simulink model "notlin2"  (Simulink 6.2)
settings: Solver=ode45  StartTime=0  StopTime=0.2
libraries: simulink x6
settings Model: Creator=Admin  LastModifiedBy=wahwat
settings OptimizationCC: BooleanDataType=off
settings HardwareCC: TargetUnknown=on

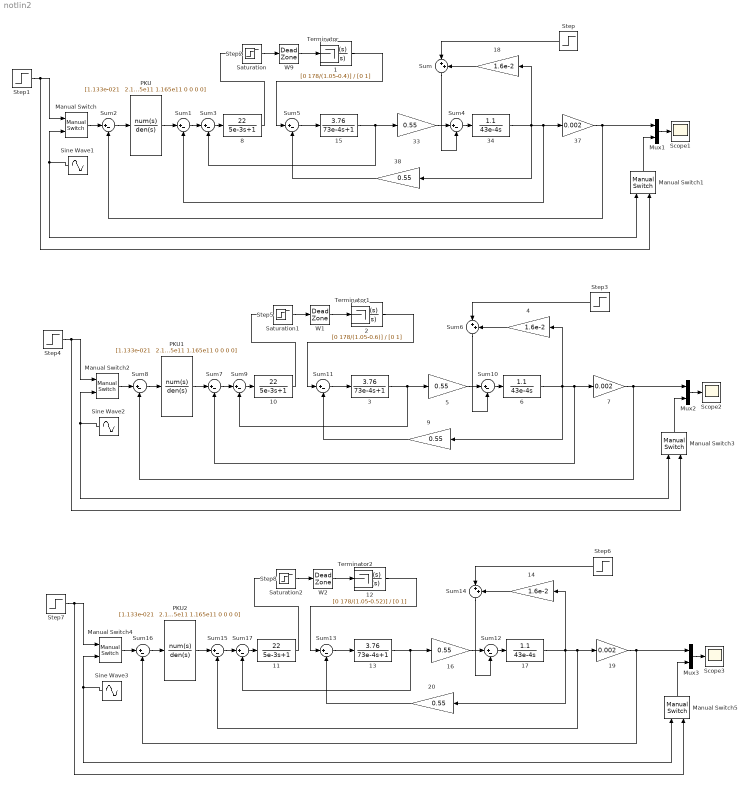
== system notlin2 ==
  1 : TransferFcn  Numerator=[0 178/(1.05-0.4)]  Denominator=[0 1]
  10 : TransferFcn  Numerator=[22]  Denominator=[5e-3 1]
  11 : TransferFcn  Numerator=[22]  Denominator=[5e-3 1]
  12 : TransferFcn  Numerator=[0 178/(1.05-0.52)]  Denominator=[0 1]
  13 : TransferFcn  Numerator=[3.76]  Denominator=[73e-4 1]
  14 : Gain  Orientation=left  Gain=1.6e-2
  15 : TransferFcn  Numerator=[3.76]  Denominator=[73e-4 1]
  16 : Gain  Gain=0.55
  17 : TransferFcn  Numerator=[1.1]  Denominator=[43e-4 0]
  18 : Gain  Orientation=left  Gain=1.6e-2
  19 : Gain  Gain=0.002
  2 : TransferFcn  Numerator=[0 178/(1.05-0.6)]  Denominator=[0 1]
  20 : Gain  Orientation=left  Gain=0.55
  3 : TransferFcn  Numerator=[3.76]  Denominator=[73e-4 1]
  33 : Gain  Gain=0.55
  34 : TransferFcn  Numerator=[1.1]  Denominator=[43e-4 0]
  37 : Gain  Gain=0.002
  38 : Gain  Orientation=left  Gain=0.55
  4 : Gain  Orientation=left  Gain=1.6e-2
  5 : Gain  Gain=0.55
  6 : TransferFcn  Numerator=[1.1]  Denominator=[43e-4 0]
  7 : Gain  Gain=0.002
  8 : TransferFcn  Numerator=[22]  Denominator=[5e-3 1]
  9 : Gain  Orientation=left  Gain=0.55
  Manual Switch : simulink/Signal Routing/Manual Switch  sw=0  action=0
  Manual Switch1 : simulink/Signal Routing/Manual Switch  Orientation=up  sw=1  action=0
  Manual Switch2 : simulink/Signal Routing/Manual Switch  sw=1  action=0
  Manual Switch3 : simulink/Signal Routing/Manual Switch  Orientation=up  sw=0  action=0
  Manual Switch4 : simulink/Signal Routing/Manual Switch  sw=1  action=0
  Manual Switch5 : simulink/Signal Routing/Manual Switch  Orientation=up  sw=0  action=0
  Mux1 : Mux  Inputs=2
  Mux2 : Mux  Inputs=2
  Mux3 : Mux  Inputs=2
  PKU : TransferFcn  Numerator="[1.133e-021   2.149e-018   7.179e-015   9.662e-12   1.32e-8   1.178e-5   0.006738 2.695 797.4 1.793e5 3.092e7 4.05e9 3.931e11 2.655e13 1.118e15 2.286e16 6.608e16 0 0 0 0]"  Denominator=[1.375e-40 2.581e-35 1.542e-30 3.734e-26 3.926e-22 1.734e-18 2.989e-15 5.009e-12 4.374e-9 2.316e-6 0.00084 0.2265 45.5 6878 7.666e5 5.962e7 2.89e9 6.806e10 2.35e11 1.165e11 0 0 0 0]
  PKU1 : TransferFcn  Numerator="[1.133e-021   2.149e-018   7.179e-015   9.662e-12   1.32e-8   1.178e-5   0.006738 2.695 797.4 1.793e5 3.092e7 4.05e9 3.931e11 2.655e13 1.118e15 2.286e16 6.608e16 0 0 0 0]"  Denominator=[1.375e-40 2.581e-35 1.542e-30 3.734e-26 3.926e-22 1.734e-18 2.989e-15 5.009e-12 4.374e-9 2.316e-6 0.00084 0.2265 45.5 6878 7.666e5 5.962e7 2.89e9 6.806e10 2.35e11 1.165e11 0 0 0 0]
  PKU2 : TransferFcn  Numerator="[1.133e-021   2.149e-018   7.179e-015   9.662e-12   1.32e-8   1.178e-5   0.006738 2.695 797.4 1.793e5 3.092e7 4.05e9 3.931e11 2.655e13 1.118e15 2.286e16 6.608e16 0 0 0 0]"  Denominator=[1.375e-40 2.581e-35 1.542e-30 3.734e-26 3.926e-22 1.734e-18 2.989e-15 5.009e-12 4.374e-9 2.316e-6 0.00084 0.2265 45.5 6878 7.666e5 5.962e7 2.89e9 6.806e10 2.35e11 1.165e11 0 0 0 0]
  Saturation : Saturate  UpperLimit=+178  LowerLimit=-178
  Saturation1 : Saturate  UpperLimit=+178  LowerLimit=-178
  Saturation2 : Saturate  UpperLimit=+178  LowerLimit=-178
  Scope1 : Scope
      settings: TickLabels=on  TimeRange=0.1
  Scope2 : Scope
      settings: TickLabels=on  TimeRange=0.1
  Scope3 : Scope
      settings: TickLabels=on  TimeRange=0.1  SaveName=ScopeData2
  Sine Wave1 : Sin  Orientation=left  Frequency=200  SampleTime=0
  Sine Wave2 : Sin  Orientation=left  Frequency=200  SampleTime=0
  Sine Wave3 : Sin  Orientation=left  Frequency=200  SampleTime=0
  Step : Step  Orientation=left  Time=0  After=1.5  SampleTime=0
  Step1 : Step  Time=0  SampleTime=0
  Step2 : Step  SampleTime=0
  Step3 : Step  Orientation=left  Time=0  After=1.5  SampleTime=0
  Step4 : Step  Time=0  SampleTime=0
  Step5 : Step  SampleTime=0
  Step6 : Step  Orientation=left  Time=0  After=1.5  SampleTime=0
  Step7 : Step  Time=0  SampleTime=0
  Step8 : Step  SampleTime=0
  Sum : Sum  Orientation=down  Inputs=|++
  Sum{1..5,7..13,15..17} (15 alike) : Sum  Inputs=|+-
  Sum14 : Sum  Orientation=down  Inputs=|++
  Sum6 : Sum  Orientation=down  Inputs=|++
  Terminator : Terminator
  Terminator1 : Terminator
  Terminator2 : Terminator
  W1 : DeadZone  LowerValue=-0.6  UpperValue=+0.6  SaturateOnIntegerOverflow=on
  W2 : DeadZone  LowerValue=-0.52  UpperValue=+0.52  SaturateOnIntegerOverflow=on
  W9 : DeadZone  LowerValue=-0.4  UpperValue=+0.4  SaturateOnIntegerOverflow=on
  wires:
  Step1/1 -> Manual Switch/1, Manual Switch1/2
  Sine Wave1/1 -> Manual Switch/2, Manual Switch1/1
  Sum5/1 -> 15/1
  15/1 -> 33/1, Sum3/2
  34/1 -> 38/1, 37/1, Sum1/2, 18/1
  38/1 -> Sum5/2
  Mux1/1 -> Scope1/1
  37/1 -> Mux1/1, Sum2/2
  Manual Switch1/1 -> Mux1/2
  Manual Switch/1 -> Sum2/1
  Sum1/1 -> Sum3/1
  Sum3/1 -> 8/1
  Sum2/1 -> PKU/1
  PKU/1 -> Sum1/1
  33/1 -> Sum4/1
  Sum4/1 -> 34/1
  18/1 -> Sum/2
  Step/1 -> Sum/1
  Sum/1 -> Sum4/2
  1/1 -> Terminator/1
  Step2/1 -> Saturation/1
  Saturation/1 -> W9/1
  W9/1 -> 1/1
  8/1 -> Sum5/1
  Step4/1 -> Manual Switch2/1, Manual Switch3/2
  Sine Wave2/1 -> Manual Switch2/2, Manual Switch3/1
  Sum11/1 -> 3/1
  3/1 -> 5/1, Sum9/2
  6/1 -> 9/1, 7/1, Sum7/2, 4/1
  9/1 -> Sum11/2
  Mux2/1 -> Scope2/1
  7/1 -> Mux2/1, Sum8/2
  Manual Switch3/1 -> Mux2/2
  Manual Switch2/1 -> Sum8/1
  Sum7/1 -> Sum9/1
  Sum9/1 -> 10/1
  Sum8/1 -> PKU1/1
  PKU1/1 -> Sum7/1
  5/1 -> Sum10/1
  Sum10/1 -> 6/1
  4/1 -> Sum6/2
  Step3/1 -> Sum6/1
  Sum6/1 -> Sum10/2
  2/1 -> Terminator1/1
  Step5/1 -> Saturation1/1
  Saturation1/1 -> W1/1
  W1/1 -> 2/1
  10/1 -> Sum11/1
  Step7/1 -> Manual Switch4/1, Manual Switch5/2
  Sine Wave3/1 -> Manual Switch4/2, Manual Switch5/1
  Sum13/1 -> 13/1
  13/1 -> 16/1, Sum17/2
  17/1 -> 20/1, 19/1, Sum15/2, 14/1
  20/1 -> Sum13/2
  Mux3/1 -> Scope3/1
  19/1 -> Mux3/1, Sum16/2
  Manual Switch5/1 -> Mux3/2
  Manual Switch4/1 -> Sum16/1
  Sum15/1 -> Sum17/1
  Sum17/1 -> 11/1
  Sum16/1 -> PKU2/1
  PKU2/1 -> Sum15/1
  16/1 -> Sum12/1
  Sum12/1 -> 17/1
  14/1 -> Sum14/2
  Step6/1 -> Sum14/1
  Sum14/1 -> Sum12/2
  12/1 -> Terminator2/1
  Step8/1 -> Saturation2/1
  Saturation2/1 -> W2/1
  W2/1 -> 12/1
  11/1 -> Sum13/1
